simulink model "cIPC_linforiginalLoad"  (R2022a)
settings: Solver=FixedStepDiscrete  StartTime=0.0  StopTime=TMax  FixedStep=DT  RelTol=1e-3
undefined symbols (not defined in the file): DiscIntNeverNeededParam, DT, Ki, optimal_azimuth_offset_rad
settings Model: Creator=jhummel  LastModifiedBy=jhummel

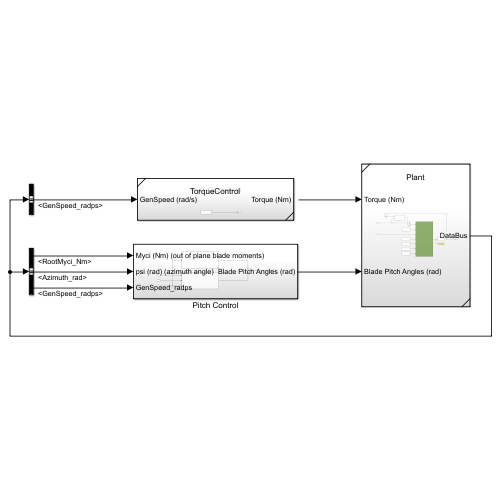
[thumbnail: Simulink's stored preview of the top-level diagram]
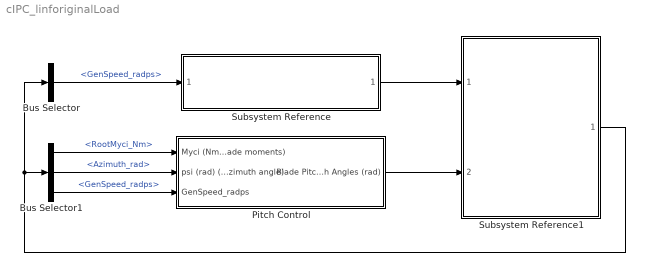
== system cIPC_linforiginalLoad ==
  Bus Selector : BusSelector  OutputSignals=GenSpeed_radps
  Bus Selector1 : BusSelector  OutputSignals=RootMyci_Nm,Azimuth_rad,GenSpeed_radps
  Pitch Control : Subsystem
  Subsystem Reference : Subsystem  ReferencedSubsystem=TorqueControl
  Subsystem Reference1 : Subsystem  ReferencedSubsystem=Plant
  wires:
  Bus Selector/1 -> Subsystem Reference/1  "<GenSpeed_radps>"
  Bus Selector1/1 -> Pitch Control/1(Myci (Nm) (out of plane blade moments))  "<RootMyci_Nm>"
  Bus Selector1/2 -> Pitch Control/2(psi (rad) (azimuth angle))  "<Azimuth_rad>"
  Bus Selector1/3 -> Pitch Control/3(GenSpeed_radps)  "<GenSpeed_radps>"
  Subsystem Reference1/1 -> Bus Selector/1, Bus Selector1/1
  Pitch Control/1(Blade Pitch Angles (rad)) -> Subsystem Reference1/2
  Subsystem Reference/1 -> Subsystem Reference1/1

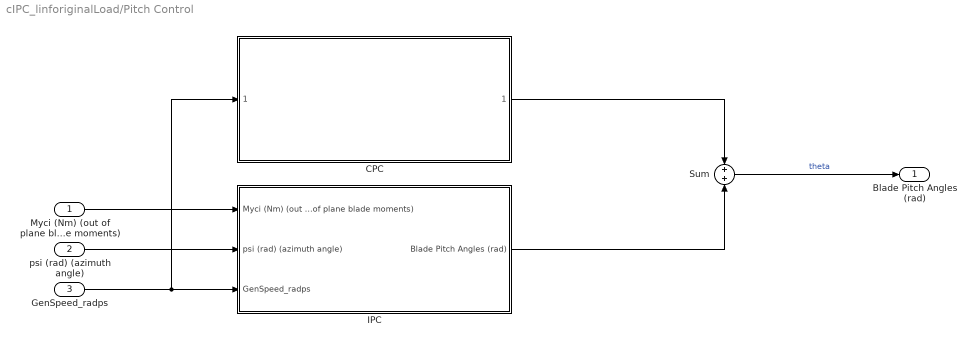
== system cIPC_linforiginalLoad/Pitch Control ==
  Myci (Nm) (out of plane blade moments) : Inport
  psi (rad) (azimuth angle) : Inport  Port=2
  GenSpeed_radps : Inport  Port=3
  CPC : Subsystem  ReferencedSubsystem=CollectivePitchControl
  IPC : Subsystem
  Sum : Sum  Inputs=+|+
  Blade Pitch Angles (rad) : Outport
  wires:
  Myci (Nm) (out of plane blade moments)/1 -> IPC/1(Myci (Nm) (out of plane blade moments))
  psi (rad) (azimuth angle)/1 -> IPC/2(psi (rad) (azimuth angle))
  GenSpeed_radps/1 -> CPC/1, IPC/3(GenSpeed_radps)
  CPC/1 -> Sum/1
  Sum/1 -> Blade Pitch Angles (rad)/1  "theta"
  IPC/1(Blade Pitch Angles (rad)) -> Sum/2

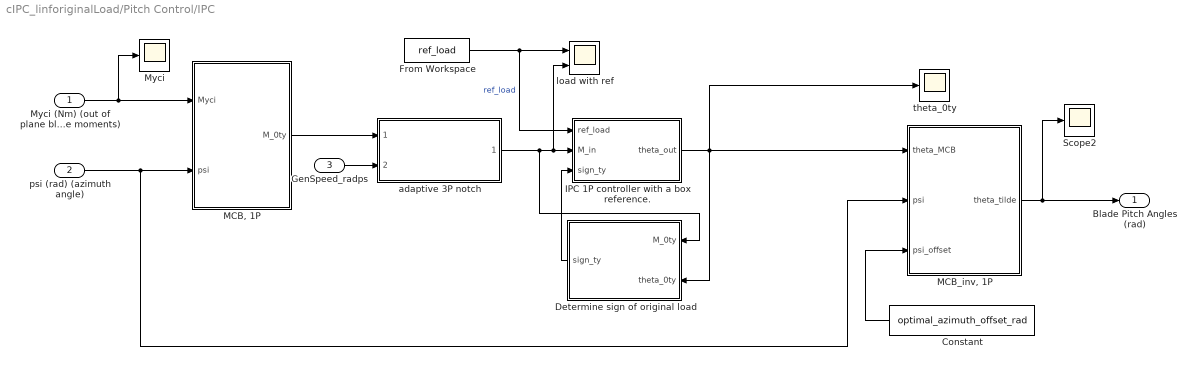
== system cIPC_linforiginalLoad/Pitch Control/IPC ==
  Myci (Nm) (out of plane blade moments) : Inport
  psi (rad) (azimuth angle) : Inport  Port=2
  GenSpeed_radps : Inport  Port=3
  Constant : Constant  Value=optimal_azimuth_offset_rad
  Determine sign of original load : Subsystem
  From Workspace : FromWorkspace  VariableName=ref_load  SampleTime=DT
  IPC 1P controller with a box reference. : Subsystem
  "MCB, 1P" : MATLAB Function  TreatAsAtomicUnit=on
  "MCB_inv, 1P" : MATLAB Function  TreatAsAtomicUnit=on
  Myci : Scope
  Scope2 : Scope
  adaptive 3P notch : Subsystem  ReferencedSubsystem=LoadFilter
  load with ref : Scope  NumInputPorts=2
  theta_0ty : Scope
  Blade Pitch Angles (rad) : Outport
  wires:
  From Workspace/1 -> load with ref/1, IPC 1P controller with a box reference./1(ref_load)  "ref_load"
  "MCB, 1P"/1(M_0ty) -> adaptive 3P notch/1
  Determine sign of original load/1(sign_ty) -> IPC 1P controller with a box reference./3(sign_ty)
  adaptive 3P notch/1 -> Determine sign of original load/1(M_0ty), load with ref/2, IPC 1P controller with a box reference./2(M_in)
  GenSpeed_radps/1 -> adaptive 3P notch/2
  "MCB_inv, 1P"/1(theta_tilde) -> Blade Pitch Angles (rad)/1, Scope2/1
  psi (rad) (azimuth angle)/1 -> "MCB_inv, 1P"/2(psi), "MCB, 1P"/2(psi)
  IPC 1P controller with a box reference./1(theta_out) -> theta_0ty/1, "MCB_inv, 1P"/1(theta_MCB), Determine sign of original load/2(theta_0ty)
  Myci (Nm) (out of plane blade moments)/1 -> Myci/1, "MCB, 1P"/1(Myci)
  Constant/1 -> "MCB_inv, 1P"/3(psi_offset)

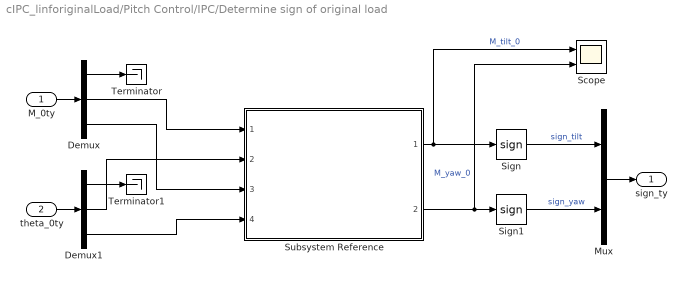
== system cIPC_linforiginalLoad/Pitch Control/IPC/Determine sign of original load ==
  M_0ty : Inport
  theta_0ty : Inport  Port=2
  Demux : Demux  Outputs=3
  Demux1 : Demux  Outputs=3
  Mux : Mux  Inputs=2
  Scope : Scope  NumInputPorts=2
  Sign : Signum
  Sign1 : Signum
  Subsystem Reference : Subsystem  ReferencedSubsystem=OriginalLoadsEstimator
  Terminator : Terminator
  Terminator1 : Terminator
  sign_ty : Outport
  wires:
  Subsystem Reference/1 -> Scope/1, Sign/1  "M_tilt_0"
  Subsystem Reference/2 -> Scope/2, Sign1/1  "M_yaw_0"
  Sign/1 -> Mux/1  "sign_tilt"
  Sign1/1 -> Mux/2  "sign_yaw"
  M_0ty/1 -> Demux/1
  theta_0ty/1 -> Demux1/1
  Demux/1 -> Terminator/1
  Demux1/1 -> Terminator1/1
  Mux/1 -> sign_ty/1
  Demux/2 -> Subsystem Reference/1
  Demux/3 -> Subsystem Reference/3
  Demux1/2 -> Subsystem Reference/2
  Demux1/3 -> Subsystem Reference/4

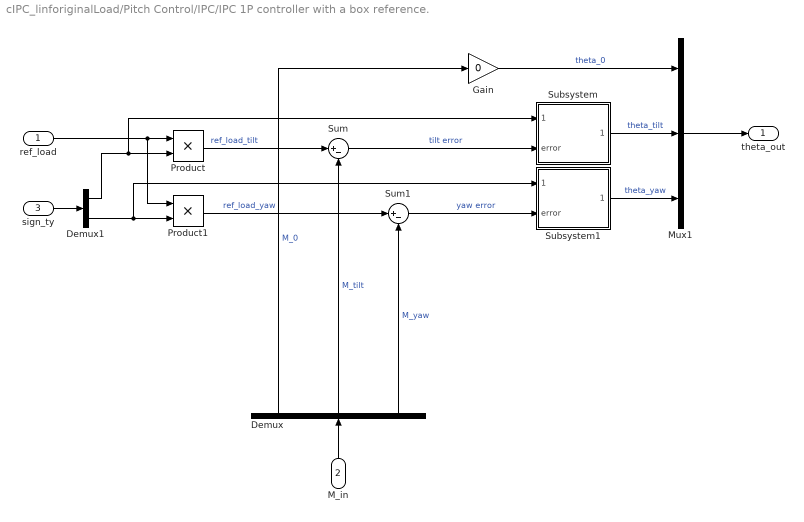
== system cIPC_linforiginalLoad/Pitch Control/IPC/IPC 1P controller with a box reference. ==
  ref_load : Inport
  M_in : Inport  Port=2
  sign_ty : Inport  Port=3
  Demux : Demux  Outputs=3
  Demux1 : Demux  Outputs=2
  Gain : Gain  Gain=0
  Mux1 : Mux  Inputs=3
  Product : Product
  Product1 : Product
  Subsystem : Subsystem
  Subsystem1 : Subsystem
  Sum : Sum  Inputs=|+-
  Sum1 : Sum  Inputs=|+-
  theta_out : Outport
  wires:
  Gain/1 -> Mux1/1  "theta_0"
  Demux/1 -> Gain/1  "M_0"
  Demux/2 -> Sum/2  "M_tilt"
  Demux/3 -> Sum1/2  "M_yaw"
  Sum/1 -> Subsystem/2(error)  "tilt error"
  Sum1/1 -> Subsystem1/2(error)  "yaw error"
  M_in/1 -> Demux/1
  Mux1/1 -> theta_out/1
  ref_load/1 -> Product/1, Product1/1
  Product/1 -> Sum/1  "ref_load_tilt"
  Product1/1 -> Sum1/1  "ref_load_yaw"
  Subsystem/1(theta_tilt) -> Mux1/2  "theta_tilt"
  Subsystem1/1(theta_yaw) -> Mux1/3  "theta_yaw"
  sign_ty/1 -> Demux1/1
  Demux1/1 -> Subsystem/1(sign_tilt), Product/2
  Demux1/2 -> Subsystem1/1(sign_yaw), Product1/2

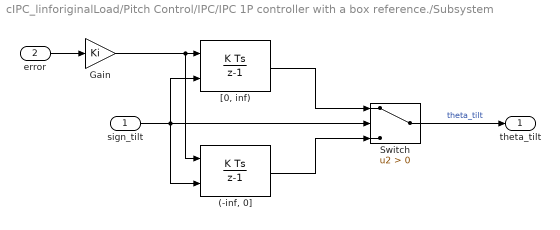
== system cIPC_linforiginalLoad/Pitch Control/IPC/IPC 1P controller with a box reference./Subsystem ==
  sign_tilt : Inport
  error : Inport  Port=2
  "(-inf, 0]" : DiscreteIntegrator  ExternalReset=either  SampleTime=-1  LimitOutput=on  UpperSaturationLimit=0  ICPrevOutput=DiscIntNeverNeededParam  ICPrevScaledInput=DiscIntNeverNeededParam
  Gain : Gain  Gain=Ki
  Switch : Switch  Criteria=u2 > Threshold  SaturateOnIntegerOverflow=off  InputSameDT=off
  "[0, inf)" : DiscreteIntegrator  ExternalReset=either  SampleTime=-1  LimitOutput=on  LowerSaturationLimit=0  ICPrevOutput=DiscIntNeverNeededParam  ICPrevScaledInput=DiscIntNeverNeededParam
  theta_tilt : Outport
  wires:
  Gain/1 -> "(-inf, 0]"/1, "[0, inf)"/1
  "[0, inf)"/1 -> Switch/1
  "(-inf, 0]"/1 -> Switch/3
  sign_tilt/1 -> "(-inf, 0]"/2, Switch/2, "[0, inf)"/2
  Switch/1 -> theta_tilt/1  "theta_tilt"
  error/1 -> Gain/1

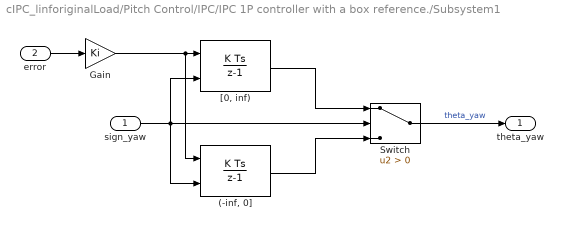
== system cIPC_linforiginalLoad/Pitch Control/IPC/IPC 1P controller with a box reference./Subsystem1 ==
  sign_yaw : Inport
  error : Inport  Port=2
  "(-inf, 0]" : DiscreteIntegrator  ExternalReset=either  SampleTime=-1  LimitOutput=on  UpperSaturationLimit=0  ICPrevOutput=DiscIntNeverNeededParam  ICPrevScaledInput=DiscIntNeverNeededParam
  Gain : Gain  Gain=Ki
  Switch : Switch  Criteria=u2 > Threshold  SaturateOnIntegerOverflow=off  InputSameDT=off
  "[0, inf)" : DiscreteIntegrator  ExternalReset=either  SampleTime=-1  LimitOutput=on  LowerSaturationLimit=0  ICPrevOutput=DiscIntNeverNeededParam  ICPrevScaledInput=DiscIntNeverNeededParam
  theta_yaw : Outport
  wires:
  Gain/1 -> "(-inf, 0]"/1, "[0, inf)"/1
  "[0, inf)"/1 -> Switch/1
  "(-inf, 0]"/1 -> Switch/3
  sign_yaw/1 -> "(-inf, 0]"/2, Switch/2, "[0, inf)"/2
  Switch/1 -> theta_yaw/1  "theta_yaw"
  error/1 -> Gain/1

== matlab function cIPC_linforiginalLoad/Pitch Control/IPC/MCB_inv, 1P ==
  data: theta_MCB input; psi input; psi_offset input; theta_tilde output
function theta_tilde = fcn(theta_MCB, psi, psi_offset)

theta_tilde = MBC_inv(theta_MCB, psi, psi_offset, 3, 1);

end

== matlab function cIPC_linforiginalLoad/Pitch Control/IPC/MCB, 1P ==
  data: Myci input; M_0ty output; psi input
function M_0ty = fcn(Myci, psi)

% Do the coordinate transformation.
M_0ty = MBC(Myci, psi, 0, 3, 1);

end
